simulink library "kl_io"  (Simulink 7.8)
settings: Solver=ode5  SolverMode=SingleTasking  StartTime=0.0  StopTime=Inf  FixedStep=0.001  RelTol=1e-3
undefined symbols (not defined in the file or in its folder): IP, TCP, TU
libraries: dec2byte x2, HvsOpen x2, Kl_RFM2G x2, CAV1553_PCI_BC x1, CAV1553B_PCI_BM x1, Rfm2g_syncRecv x1, Rfm2g_init x1, Rfm2g_syncSend x1, serial_control_ps3510 x1, serial_ps3510_recv x1, serial_send_ps3510 x1, ks_ethernet_init x1
settings Model: Creator=Administrator  LastModifiedBy=KLJS168

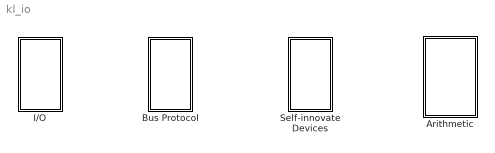
== system kl_io ==
  Arithmetic : Subsystem
  Bus Protocol : Subsystem
  I/O : Subsystem
  Self-innovate Devices : Subsystem

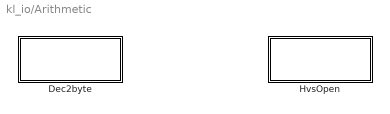
== system kl_io/Arithmetic ==
  Dec2byte : Subsystem
  HvsOpen : Subsystem

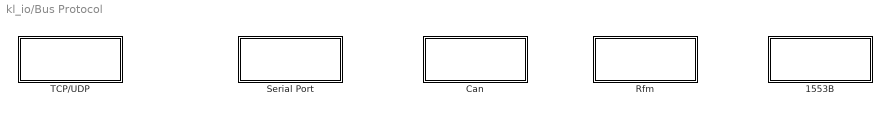
== system kl_io/Bus Protocol ==
  1553B : Subsystem
  Can : Subsystem
  Rfm : Subsystem
  Serial Port : Subsystem
  TCP/UDP : Subsystem

== system kl_io/I/O ==
  NI : Subsystem

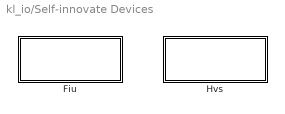
== system kl_io/Self-innovate Devices ==
  Fiu : Subsystem
  Hvs : Subsystem

== system kl_io/Arithmetic/Dec2byte ==
  note: dec2byte
      | 可将给定的 8*1 数据a 按 BIT 组成一个数据b
      | 数据a只能给值 0 或者 1
  dec : dec2byte/dec
  dec2byte : dec2byte/dec2byte
  wires:
  dec/1 -> dec2byte/1

== system kl_io/Arithmetic/HvsOpen ==
  note: 高压模拟器控制数据组包
      | 1、RELAY中constant只能给值 0 或者 1
      | 2、将 ConfData 与 Active 输出口分别接到两个 UDP 的发送端
      | 3、在线控制时只需要改变 RELAY 的值,DATAPCK不需要做任何改动
      | 4、RELAY 具体含义见硬件相关文档说明
  DATAPACK : HvsOpen/DATAPACK
  RELAY : HvsOpen/RELAY
  wires:
  RELAY/1 -> DATAPACK/1

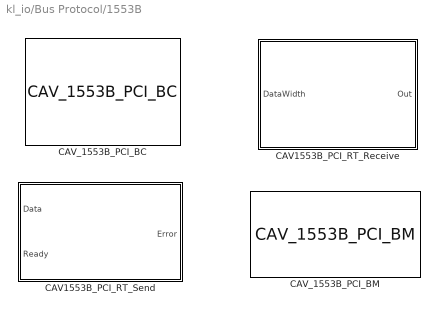
== system kl_io/Bus Protocol/1553B ==
  CAV1553B_PCI_RT_Receive : Subsystem  mask(CAV_1553B_PCI RT Receive){pci_id=0, chan_id=0, bfirst=1, sourcert_add=0, sourcert_subadd=0}
      mask prompts: pci_id "PCI ID"; chan_id "Channel ID"; bfirst "First Use"; sourcert_add "Remote Terminal:"; sourcert_subadd "Sub address:"
      mask help: This block is used for RT to receive message .
      mask init:
      | displayblock=sprintf('\n CAV 1553B RT Rece\nPCI Id: %d\nChannel Id: %d\nRT Add: %d\nSub RT: %d\n', pci_id, chan_id,sourcert_add,sourcert_subadd);
      mask StyleString: edit,edit,popup(1|2),edit,edit
      mask CallbackString:
      | ||bfir = get_param(gcb,'bfirst');
      | 
      | if(strcmp(bfir,'1')),
      |     set_param(gcb,'MaskEnables',{'on';'on';'off';'on';'on'}),
      | else
      |     set_param(gcb,'MaskEnables',{'on';'on';'off';'on';'on'}),
      | end
      | ||
      mask Display: disp(displayblock);
  CAV1553B_PCI_RT_Send : Subsystem  mask(CAV_1553B_PCI RT Send){pci_id=0, chan_id=0, bfirst=1, sourcert_add=0, sourcert_subadd=0}
      mask prompts: pci_id "PCI ID"; chan_id "Channel ID"; bfirst "First Use"; sourcert_add "Remote Terminal"; sourcert_subadd "Sub-Address"
      mask help: This block is used for RT to send messages .
      mask init:
      | displayblock=sprintf('\n1553B RT Send\nPCI Id: %d\nChannel Id: %d\nRT Add: %d\nSub RT: %d\n', pci_id, chan_id,sourcert_add,sourcert_subadd);
      mask StyleString: edit,edit,popup(1|2),edit,edit
      mask CallbackString:
      | ||bfir = get_param(gcb,'bfirst');
      | 
      | if(strcmp(bfir,'1')),
      |     set_param(gcb,'MaskEnables',{'on';'on';'off';'on';'on'}),
      | else
      |     set_param(gcb,'MaskEnables',{'on';'on';'off';'on';'on'}),
      | end
      | ||
      mask Display: disp(displayblock);
  CAV_1553B_PCI_BC : CAV1553_PCI_BC/CAV_1553B_PCI_BC  pci_id=0  chan_id=0  bc_identifer=0  bc_num=1  bus_ctrl_op=BCRT  bus_num=Bus A  sourcert_add=0  sourcert_subadd=0  destrt_add=0  destrt_subadd=0  last_bc=0  is_first_bc=0
  CAV_1553B_PCI_BM : CAV1553B_PCI_BM/CAV_1553B_PCI_BM  pci_id=0  chan_id=0  IsAllMonitor=Select Some  sourcert_add=[0]  sourcert_subadd=[0]  tr=0  NumOfMesg=1000  rev0=20  rev1=0  rev2=0

== system kl_io/Bus Protocol/Can ==

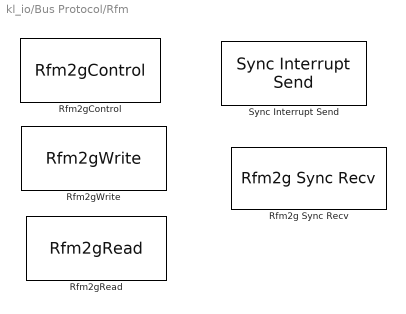
== system kl_io/Bus Protocol/Rfm ==
  Rfm2g Sync Recv : Rfm2g_syncRecv/Rfm2g Sync Recv  nodeid=0  eventtype=RFM2GEVENT_INTR1  rev0=10  rev1=0
  Rfm2gControl : Rfm2g_init/Rfm2gControl  nodeid=0  rev0=0  rev1=0
  Rfm2gRead : Kl_RFM2G/Rfm2gRead  ReadNodeId=0  ReadBufSize=100  ReadOffset=100
  Rfm2gWrite : Kl_RFM2G/Rfm2gWrite  WriteNodeId=0  WriteBufSize=100  WriteOffset=100
  Sync Interrupt Send : Rfm2g_syncSend/Sync Interrupt Send  nodeid=0  towhich=1  eventtype=RFM2GEVENT_INTR1  rev0=0  rev1=0

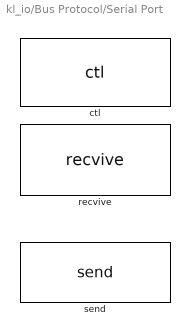
== system kl_io/Bus Protocol/Serial Port ==
  ctl : serial_control_ps3510/ctl  choosewrongdata=TU-5011  ctlid=1  resv0=0  resv1=0  sendchl=1  resv2=Send  lenbit=Data8  paritybit=Odd  baud=9600  resv3=500000  stopbit=1  parityenbale=DIS  mode=RS232
  recvive : serial_ps3510_recv/recvive  ctlid=TU-5011  resv0=0  resv1=0  recvchl=1  resv2=0  resv3=0
  send : serial_send_ps3510/send  ctlid=TU-5011  resv1=0  resv2=0  resv0=1  resv3=0

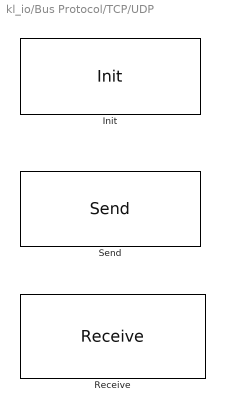
== system kl_io/Bus Protocol/TCP/UDP ==
  Init : ks_ethernet_init/Init  ctl_id=1  l_addr=[0 0 0 0]  l_port=0  r_para0=UDP  r_para4=NonBlocking  r_para3=0  r_para1=[192 168 1 100]  r_para2=10000
  Receive : ks_ethernet_recv/Receive  ctl_id=1  protocol=UDP  isBcast=off  src_addr=[0 0 0 0]  src_port=0  enRecvTh=Disable  r_para0=100  r_para1=No  r_para2=[224 225 226 227]  r_para3=[0 0 0 0]  r_para4=0
  Send : ks_ethernet_send/Send  ctl_id=1  protocol=UDP  isBcast=off  dst_addr=[192 168 1 100]  dst_port=10000  r_para0=0  r_para1=0  r_para2=0  r_para3=0  r_para4=0

== system kl_io/I/O/NI ==
  DAQ : Subsystem

== system kl_io/Self-innovate Devices/Fiu ==
  KLFIUDATA : KL_FaultInsertUnit_v2_1/KLFIUDATA  nContrId=0  nRev1=[192 168 1 6]  nRev2=50099  nRev0=0  nWorkMode=0  nCanSendId=0  nCanRecvId=0  nPinNum=[0]  nActionNum=[10]  nWithLoad=[0]

== system kl_io/Self-innovate Devices/Hvs ==
  KL HVS CTL : KL_HignVoltageSimuCtl/KL HVS CTL  CtlId=0  rev0=TCP/IP  DestIp=[192 168 2 240]  DestPort=2040  rev1=1  rev2=1  rev3=0  rev4=0

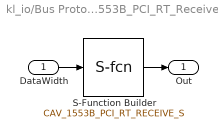
== system kl_io/Bus Protocol/1553B/CAV1553B_PCI_RT_Receive ==
  DataWidth : Inport
  S-Function Builder : S-Function  InitFcn=try, set_param(gcb,'FunctionName','CAV_1553B_PCI_RT_RECEIVE_S'), end  FunctionName=CAV_1553B_PCI_RT_RECEIVE_S  Parameters=pci_id,chan_id,bfirst,sourcert_add,sourcert_subadd  EnableBusSupport=off  mask(S-Function Builder){}
      mask help: The S-Function Builder block creates a wrapper C-MEX S-function from your supplied C code with multiple input ports, output ports, and a variable number of scalar, vector, or matrix parameters. The input and output ports can propagate Simulink built-in data types, fixed-point datatypes, complex, frame, 1-D, and 2-D signals. This block also supports discrete and continuous states of type real. You can optionally have the block generate a TLC file to be used with Real-Time Workshop for code generation.
      mask init:
      | val = [[.9  0.75 0.75 1 1 .9 .9 1]',[1 1 0.75 0.75 .9 .9 1 .9]'];try , sys = get_param(gcb,'SfunBuilderFcnName');if isempty(sys), sys = get_param(gcb,'FunctionName'); end,catch, sys = get_param(gcb,'FunctionName'); end
      settings: CopyFcn=set_param(gcbh,'LinkStatus','none')  PreSaveFcn=try, set_param(gcb,'FunctionName','CAV_1553B_PCI_RT_RECEIVE_S'), end  OpenFcn=sfunctionwizard(gcbh)
      mask Display: plot(val(:,1),val(:,2)),disp(sys)port_label('input',1,'u0')port_label('output',1,'y0')
  Out : Outport
  wires:
  DataWidth/1 -> S-Function Builder/1
  S-Function Builder/1 -> Out/1

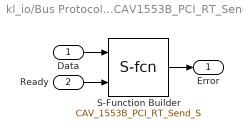
== system kl_io/Bus Protocol/1553B/CAV1553B_PCI_RT_Send ==
  Data : Inport
  Ready : Inport  Port=2
  S-Function Builder : S-Function  InitFcn=try, set_param(gcb,'FunctionName','CAV_1553B_PCI_RT_Send_S'), end  FunctionName=CAV_1553B_PCI_RT_Send_S  Parameters=pci_id,chan_id,bfirst,sourcert_add,sourcert_subadd  WizardData=DataTag0  EnableBusSupport=off  mask(S-Function Builder){}
      mask help: The S-Function Builder block creates a wrapper C-MEX S-function from your supplied C code with multiple input ports, output ports, and a variable number of scalar, vector, or matrix parameters. The input and output ports can propagate Simulink built-in data types, fixed-point datatypes, complex, frame, 1-D, and 2-D signals. This block also supports discrete and continuous states of type real. You can optionally have the block generate a TLC file to be used with Real-Time Workshop for code generation.
      mask init: same as kl_io/Bus Protocol/1553B/CAV1553B_PCI_RT_Receive/S-Function Builder
      settings: CopyFcn=set_param(gcbh,'LinkStatus','none')  PreSaveFcn=try, set_param(gcb,'FunctionName','CAV_1553B_PCI_RT_Send_S'), end  OpenFcn=sfunctionwizard(gcbh)
      mask Display: plot(val(:,1),val(:,2)),disp(sys)port_label('input',1,'u0')port_label('input',2,'u1')port_label('output',1,'y0')
  Error : Outport
  wires:
  Data/1 -> S-Function Builder/1
  S-Function Builder/1 -> Error/1
  Ready/1 -> S-Function Builder/2

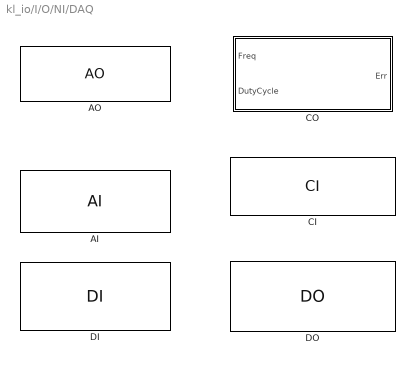
== system kl_io/I/O/NI/DAQ ==
  AI : NI_Board_AI/AI  nCon=0  nDev=1  nChan=0  nMode=DAQmx_Val_RSE  nMax=10  nMin=-10  nSamp=0  nReserve=0
  AO : NI_Board_AO/AO  nCon=0  nDev=1  nChan=[1]  nMax=10  nMin=-10  nSample=Voltage  nReserve=0
  CI : NiCiDuty/CI  devid=0  chanid=0
  CO : Subsystem  mask(NI_PCI_6289 For Counter Output){nDev=0, nChan=0, initialDelay=0}
      mask prompts: nDev "Dev ID:"; nChan "Chan ID:"; initialDelay "Delay Time:"
      mask help:
      | This block is used for CO.
      | You can specify the counter which you want to use.
      |
      | Block Parameters
      | Dev ID
      |     You can find the ID by nilsdev commond after you install DAQmx.
      | Chan ID
      |     Specify counter which you want to use.
      | Delay Time
      |     The amount of time in seconds to wait before generating the first pulse.
      | Err
      |     It will be -1 when a error occur.
      | DutyCycle
      |     The width of the pulse divided by the pulse period .
      | Freq
      |     The frequency at which to generate pulses .
      mask init:
      | displayblock=sprintf('\nCO Frequency\nDev ID: %d Chan ID: %d\nDelay Time: %.2f\n', nDev, nChan,initialDelay);
      mask Help: You must Install The DAQmx of NI before you use it.You can find in Driver Dir.And there is a INSTALL file that will help you install it.
      mask Display: disp(displayblock);
  DI : KL_SimuDI/DI  nDev=1  nPort=1  nLine=0  nLineSelect=MultiLine  nStartLine=0  nEndLine=7
  DO : KL_SimuDO/DO  nDev=1  nPort=1  nLine=0  nLineSelect=MultiLine  nStartLine=0  nEndLine=7

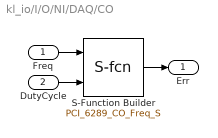
== system kl_io/I/O/NI/DAQ/CO ==
  Freq : Inport
  DutyCycle : Inport  Port=2
  S-Function Builder : S-Function  InitFcn=try, set_param(gcb,'FunctionName','PCI_6289_CO_Freq_S'), end  FunctionName=PCI_6289_CO_Freq_S  Parameters=nDev,nChan,initialDelay  WizardData=DataTag1  EnableBusSupport=off  mask(S-Function Builder){}
      mask help: The S-Function Builder block creates a wrapper C-MEX S-function from your supplied C code with multiple input ports, output ports, and a variable number of scalar, vector, or matrix parameters. The input and output ports can propagate Simulink built-in data types, fixed-point datatypes, complex, frame, 1-D, and 2-D signals. This block also supports discrete and continuous states of type real. You can optionally have the block generate a TLC file to be used with Real-Time Workshop for code generation.
      mask init: same as kl_io/Bus Protocol/1553B/CAV1553B_PCI_RT_Receive/S-Function Builder
      settings: CopyFcn=set_param(gcbh,'LinkStatus','none')  PreSaveFcn=try, set_param(gcb,'FunctionName','PCI_6289_CO_Freq_S'), end  OpenFcn=sfunctionwizard(gcbh)
      mask Display: plot(val(:,1),val(:,2)),disp(sys)port_label('input',1,'u0')port_label('input',2,'u1')port_label('output',1,'y0')
  Err : Outport
  wires:
  DutyCycle/1 -> S-Function Builder/2
  S-Function Builder/1 -> Err/1
  Freq/1 -> S-Function Builder/1
